simulink model "gm_uz_pmsm_model_9ph_21b_all_double_vnl"  (R2021b)
settings: Solver=FixedStepDiscrete  StartTime=0.0  StopTime=0.8  RelTol=1e-3
PreLoadFcn:
  | uz_pmsm_model_9ph_init_parameter
undefined symbols (not defined in the file or in its folder): a, b, c, friction_coefficient, inertia, k_i_d, k_i_q, k_p_d, k_p_q, Kpd, L_d, L_o1, L_o2, L_q, L_x1, L_x2, L_y1, L_y2, L_zero, polepair, psi_pm, R_1, static_friction_torque, Tnd, ts
libraries: hdlmdlgenlib x139, hdlsllib x90, dspsigops x21, simulink x17, slpidlib x2, spsAlphaBetaZerotodq0Lib x1, pid_lib x1, spsdq0toAlphaBetaZeroLib x1
(part 3 of 5)

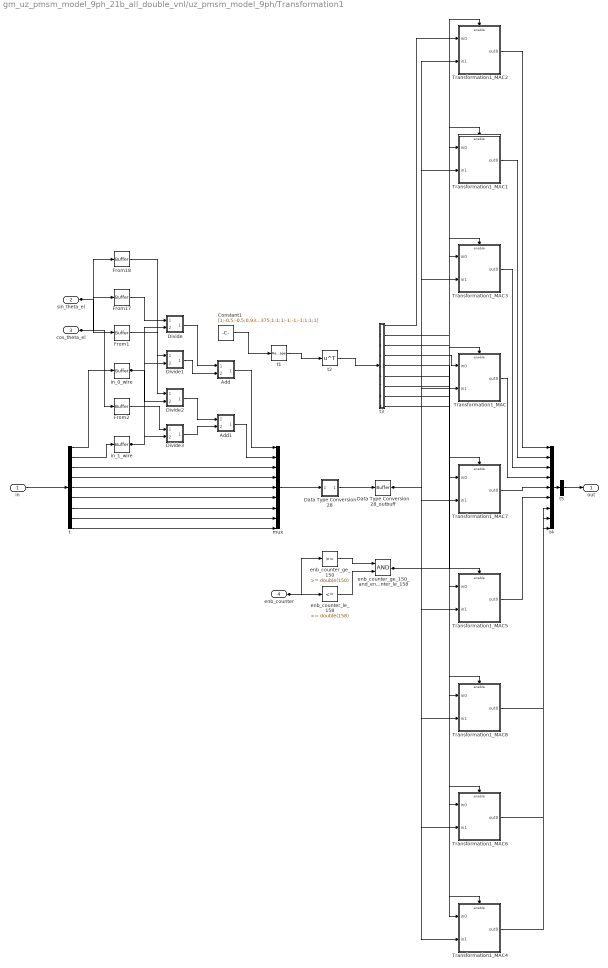
== system gm_uz_pmsm_model_9ph_21b_all_double_vnl/uz_pmsm_model_9ph/Transformation1 ==
  in : Inport  OutDataTypeStr=single  PortDimensions=[9]  SampleTime=1e-08
  sin_theta_el : Inport  Port=2  OutDataTypeStr=single  SampleTime=1e-08
  cos_theta_el : Inport  Port=3  OutDataTypeStr=single  SampleTime=1e-08
  enb_counter : Inport  Port=4  OutDataTypeStr=uint8  SampleTime=1e-08
  Add : Subsystem
      mask Display: disp('NFP\nadd');
  Add1 : Subsystem
      mask Display: disp('NFP\nadd');
  Constant1 : Constant  Value=[1;-0.5;-0.5;0.939697265625;-0.7660369873046875;-0.17364501953125;0.7660369873046875;-0.939697265625;0.17364501953125;0;0.86602783203125;-0.86602783203125;0.3420257568359375;0.642791748046875;-0.98480224609375;0.642791748046875;0.3420257568359375;-0.98480224609375;1;1;1;0.5;0.5;0.5;-0.5;-0.5;-0.5;0;0;0;0.86602783203125;0.86602783203125;0.86602783203125;0.86602783203125;0.86602783203125;0.86602783203125;1;-0.5;-0.5;-0.17364501953125;0.939697265625;-0.7660369873046875;-0.939697265625;0.17364501953125;0.7660369873046875;0;-0.86602783203125;0.86602783203125;0.98480224609375;-0.3420257568359375;-0.642791748046875;-0.3420257568359375;0.98480224609375;-0.642791748046875;1;-0.5;-0.5;-0.7660369873046875;-0.17364501953125;0.939697265625;0.17364501953125;0.7660369873046875;-0.939697265625;0;0.86602783203125;-0.86602783203125;0.642791748046875;-0.98480224609375;0.3420257568359375;-0.98480224609375;0.642791748046875;0.3420257568359375;1;1;1;-1;-1;-1;1;1;1]  OutDataTypeStr=fixdt(1, 18, 16)  SampleTime=1e-08
  Data Type Conversion28 : Subsystem
      mask Display: disp('NFP\nconv');
  Data Type Conversion28_outbuff : hdlmdlgenlib/Buffer
      settings: SourceProductBaseCode=SL
  Divide : Subsystem
      mask Display: disp('NFP\nmul');
  Divide1 : Subsystem
      mask Display: disp('NFP\nmul');
  Divide2 : Subsystem
      mask Display: disp('NFP\nmul');
  Divide3 : Subsystem
      mask Display: disp('NFP\nmul');
  From{1..2,17..18} (4 alike) : hdlmdlgenlib/Buffer
      settings: SourceProductBaseCode=SL
  Transformation1_MAC : Subsystem
      settings: MinAlgLoopOccurrences=on
  Transformation1_MAC1 : Subsystem
      settings: MinAlgLoopOccurrences=on
  Transformation1_MAC2 : Subsystem
      settings: MinAlgLoopOccurrences=on
  Transformation1_MAC3 : Subsystem
      settings: MinAlgLoopOccurrences=on
  Transformation1_MAC4 : Subsystem
      settings: MinAlgLoopOccurrences=on
  Transformation1_MAC5 : Subsystem
      settings: MinAlgLoopOccurrences=on
  Transformation1_MAC6 : Subsystem
      settings: MinAlgLoopOccurrences=on
  Transformation1_MAC7 : Subsystem
      settings: MinAlgLoopOccurrences=on
  Transformation1_MAC8 : Subsystem
      settings: MinAlgLoopOccurrences=on
  enb_counter_ge_150 : simulink/Logic and Bit Operations/Compare To Constant  relop=>=  const=double(150)  OutDataTypeStr=boolean
  enb_counter_ge_150_and_enb_counter_le_158 : Logic  AllPortsSameDT=off  OutDataTypeStr=boolean  SampleTime=1e-08
  enb_counter_le_158 : simulink/Logic and Bit Operations/Compare To Constant  relop=<=  const=double(158)  OutDataTypeStr=boolean
  in_0_wire : hdlmdlgenlib/Buffer
      settings: SourceProductBaseCode=SL
  in_1_wire : hdlmdlgenlib/Buffer
      settings: SourceProductBaseCode=SL
  mux : Mux  Inputs=9
  t : Demux  Outputs=9
  t1 : Reshape  OutputDimensionality=Customize  OutputDimensions=[9,9]
  t2 : Math  Operator=transpose  SaturateOnIntegerOverflow=on
  t3 : Subsystem
  t4 : Mux  Inputs=9
  t5 : Concatenate  NumInputs=1  Mode=Multidimensional array  ConcatenateDimension=2
  out : Outport  SampleTime=1e-08
  wires:
  enb_counter/1 -> enb_counter_ge_150/1, enb_counter_le_158/1
  cos_theta_el/1 -> From17/1, From2/1
  sin_theta_el/1 -> From1/1, From18/1
  in/1 -> t/1
  enb_counter_le_158/1 -> enb_counter_ge_150_and_enb_counter_le_158/2
  enb_counter_ge_150/1 -> enb_counter_ge_150_and_enb_counter_le_158/1
  enb_counter_ge_150_and_enb_counter_le_158/1 -> Transformation1_MAC4/Enable, Transformation1_MAC6/Enable, Transformation1_MAC8/Enable, Transformation1_MAC5/Enable, Transformation1_MAC7/Enable, Transformation1_MAC/Enable, Transformation1_MAC3/Enable, Transformation1_MAC1/Enable, Transformation1_MAC2/Enable
  t3/9(out8) -> Transformation1_MAC4/1(in0)
  t3/8(out7) -> Transformation1_MAC6/1(in0)
  t3/7(out6) -> Transformation1_MAC8/1(in0)
  t3/6(out5) -> Transformation1_MAC5/1(in0)
  t3/5(out4) -> Transformation1_MAC7/1(in0)
  t3/4(out3) -> Transformation1_MAC/1(in0)
  t3/3(out2) -> Transformation1_MAC3/1(in0)
  t3/2(out1) -> Transformation1_MAC1/1(in0)
  t3/1(out0) -> Transformation1_MAC2/1(in0)
  Divide3/1(Out1) -> Add1/2(In2)
  Divide2/1(Out1) -> Add1/1(In1)
  Divide1/1(Out1) -> Add/2(In2)
  Divide/1(Out1) -> Add/1(In1)
  Data Type Conversion28/1(Out1) -> Data Type Conversion28_outbuff/1
  Add1/1(Out1) -> mux/2
  Add/1(Out1) -> mux/1
  t4/1 -> t5/1
  Transformation1_MAC4/1(out0) -> t4/9
  Transformation1_MAC6/1(out0) -> t4/8
  Transformation1_MAC8/1(out0) -> t4/7
  Transformation1_MAC5/1(out0) -> t4/6
  Transformation1_MAC7/1(out0) -> t4/5
  Transformation1_MAC/1(out0) -> t4/4
  Transformation1_MAC3/1(out0) -> t4/3
  Transformation1_MAC1/1(out0) -> t4/2
  Transformation1_MAC2/1(out0) -> t4/1
  t2/1 -> t3/1(in0)
  Constant1/1 -> t1/1
  t/9 -> mux/9
  t/8 -> mux/8
  t/7 -> mux/7
  t/6 -> mux/6
  t/5 -> mux/5
  t/4 -> mux/4
  t/3 -> mux/3
  t/2 -> in_1_wire/1
  t/1 -> in_0_wire/1
  mux/1 -> Data Type Conversion28/1(In1)
  t5/1 -> out/1
  From2/1 -> Divide3/1(In1)
  From18/1 -> Divide1/1(In1)
  From17/1 -> Divide/1(In1)
  From1/1 -> Divide2/1(In1)
  in_1_wire/1 -> Divide1/2(In2), Divide3/2(In2)
  in_0_wire/1 -> Divide/2(In2), Divide2/2(In2)
  Data Type Conversion28_outbuff/1 -> Transformation1_MAC4/2(in1), Transformation1_MAC6/2(in1), Transformation1_MAC8/2(in1), Transformation1_MAC5/2(in1), Transformation1_MAC7/2(in1), Transformation1_MAC/2(in1), Transformation1_MAC3/2(in1), Transformation1_MAC1/2(in1), Transformation1_MAC2/2(in1)
  t1/1 -> t2/1

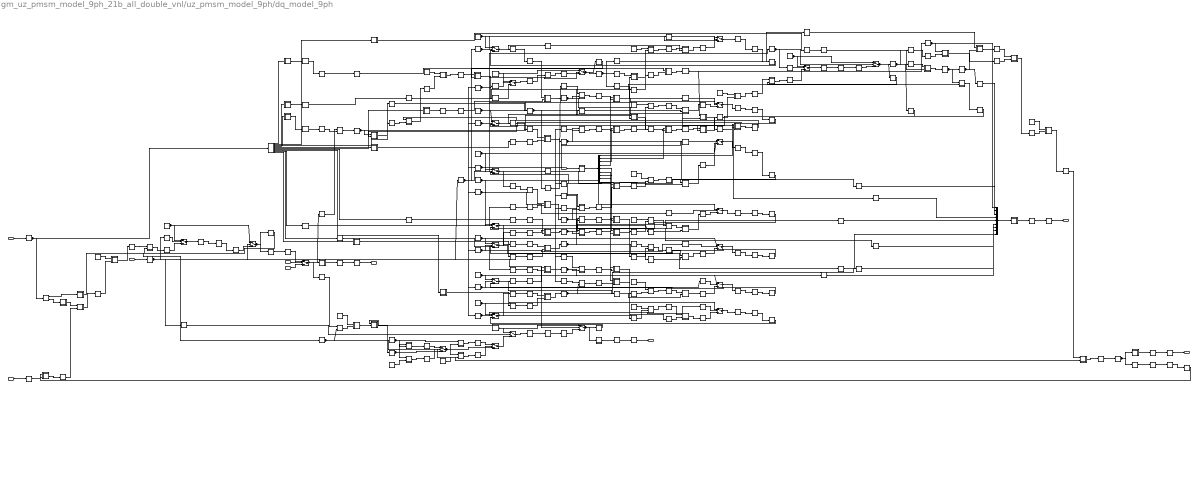
== system gm_uz_pmsm_model_9ph_21b_all_double_vnl/uz_pmsm_model_9ph/dq_model_9ph ==
  note: This signal introduces an algebraic loop if simulate_mechanical is true!
  note: PMSM electric and magentic
  note: Mechanical
  note: o1 equation
  note: DQ equations
  note: o2 equation
  note: x1 equation
  note: y1 equation
  note: x2 equation
  note: y2 equation
  note: zero equation
  note: load torque negative!!!
  note: https://de.mathworks.com/help/releases/R2021a/hdlcoder/ug/troubleshoot-generate-implementation-model-from-simscape-pmsm.html?searchHighlight=troubleshoot-generate-implementation-model-from-simscape-pmsm&s_tid=doc_srchtitle
  load_torque : Inport  OutDataTypeStr=single  PortDimensions=1  SampleTime=1e-08
  <reset_integrators> : Inport  Port=2  OutDataTypeStr=boolean  PortDimensions=1  SampleTime=1e-08
  <simulate_mechanical> : Inport  Port=3  OutDataTypeStr=boolean  PortDimensions=1  SampleTime=1e-08
  omega_mech : Inport  Port=4  OutDataTypeStr=single  PortDimensions=1  SampleTime=1e-08
  voltage_input_dq : Inport  Port=5  OutDataTypeStr=single  PortDimensions=[9]  SampleTime=1e-08
  physical_parameters : Inport  Port=6  SampleTime=2e-06
  Add : Subsystem
      mask Display: disp('NFP\nadd');
  Add1 : Subsystem
      mask Display: disp('NFP\nadd');
  Add1_outbuff : hdlmdlgenlib/Buffer
      settings: SourceProductBaseCode=SL
  Add2 : Subsystem
      mask Display: disp('NFP\nadd');
  Add2_outbuff : hdlmdlgenlib/Buffer
      settings: SourceProductBaseCode=SL
  Add3 : Subsystem
      mask Display: disp('NFP\nadd');
  Add3_outbuff : hdlmdlgenlib/Buffer
      settings: SourceProductBaseCode=SL
  Add4 : Subsystem
      mask Display: disp('NFP\nadd');
  Add4_outbuff : hdlmdlgenlib/Buffer
      settings: SourceProductBaseCode=SL
  Add5 : Subsystem
      mask Display: disp('NFP\nadd');
  Add5_outbuff : hdlmdlgenlib/Buffer
      settings: SourceProductBaseCode=SL
  Add6 : Subsystem
      mask Display: disp('NFP\nadd');
  Add6_outbuff : hdlmdlgenlib/Buffer
      settings: SourceProductBaseCode=SL
  Add_outbuff : hdlmdlgenlib/Buffer
      settings: SourceProductBaseCode=SL
  Compare To Constant1_const : Constant  Value=double(-3.1415927410125732)  OutDataTypeStr=double  SampleTime=1e-08
  Compare To Constant1_relop : Subsystem
      mask Display: disp('NFP\nrelop');
  Compare To Constant1_relop_outbuff : hdlmdlgenlib/Buffer
      settings: SourceProductBaseCode=SL
  Compare To Constant_const : Constant  Value=double(3.1415927410125732)  OutDataTypeStr=double  SampleTime=1e-08
  Compare To Constant_relop : Subsystem
      mask Display: disp('NFP\nrelop');
  Compare To Constant_relop_outbuff : hdlmdlgenlib/Buffer
      settings: SourceProductBaseCode=SL
  Constant : Constant  Value=double(6.283185307179586)  OutDataTypeStr=double  SampleTime=1e-08
  Data Type Conversion : Subsystem
      mask Display: disp('NFP\nconv');
  Data Type Conversion1 : Subsystem
      mask Display: disp('NFP\nconv');
  Data Type Conversion10 : Subsystem
      mask Display: disp('NFP\nconv');
  Data Type Conversion11 : Subsystem
      mask Display: disp('NFP\nconv');
  Data Type Conversion12 : Subsystem
      mask Display: disp('NFP\nconv');
  Data Type Conversion13 : Subsystem
      mask Display: disp('NFP\nconv');
  Data Type Conversion1_outbuff : hdlmdlgenlib/Buffer
      settings: SourceProductBaseCode=SL
  Data Type Conversion2 : Subsystem
      mask Display: disp('NFP\nconv');
  Data Type Conversion21 : Subsystem
      mask Display: disp('NFP\nconv');
  Data Type Conversion3 : Subsystem
      mask Display: disp('NFP\nconv');
  Data Type Conversion31 : Subsystem
      mask Display: disp('NFP\nconv');
  Data Type Conversion4 : Subsystem
      mask Display: disp('NFP\nconv');
  Data Type Conversion41 : Subsystem
      mask Display: disp('NFP\nconv');
  Data Type Conversion4_outbuff : hdlmdlgenlib/Buffer
      settings: SourceProductBaseCode=SL
  Data Type Conversion5 : Subsystem
      mask Display: disp('NFP\nconv');
  Data Type Conversion51 : Subsystem
      mask Display: disp('NFP\nconv');
  Data Type Conversion6 : Subsystem
      mask Display: disp('NFP\nconv');
  Data Type Conversion61 : Subsystem
      mask Display: disp('NFP\nconv');
  Data Type Conversion7 : Subsystem
      mask Display: disp('NFP\nconv');
  Data Type Conversion71 : Subsystem
      mask Display: disp('NFP\nconv');
  Data Type Conversion8 : Subsystem
      mask Display: disp('NFP\nconv');
  Data Type Conversion9 : Subsystem
      mask Display: disp('NFP\nconv');
  Delay : RateTransition  OutPortSampleTimeOpt=Multiple of input port sample time  OutPortSampleTimeMultiple=200
  Delay1 : RateTransition  OutPortSampleTimeOpt=Multiple of input port sample time  OutPortSampleTimeMultiple=200
  Delay1_lowered{,1..10} (11 alike) : RateTransition  OutPortSampleTimeOpt=Multiple of input port sample time  OutPortSampleTimeMultiple=200
  Delay2 : RateTransition  OutPortSampleTimeOpt=Multiple of input port sample time  OutPortSampleTimeMultiple=200
  Divide : Subsystem
      mask Display: disp('NFP\nmul');
  Divide1 : Subsystem
      mask Display: disp('NFP\nmul');
  Divide10 : Subsystem
      mask Display: disp('NFP\nmul');
  Divide10_outbuff : hdlmdlgenlib/Buffer
      settings: SourceProductBaseCode=SL
  Divide11 : Subsystem
      mask Display: disp('NFP\nmul');
  Divide11_outbuff : hdlmdlgenlib/Buffer
      settings: SourceProductBaseCode=SL
  Divide12 : Subsystem
      mask Display: disp('NFP\nmul');
  Divide12_outbuff : hdlmdlgenlib/Buffer
      settings: SourceProductBaseCode=SL
  Divide13 : Subsystem
      mask Display: disp('NFP\nmul');
  Divide13_outbuff : hdlmdlgenlib/Buffer
      settings: SourceProductBaseCode=SL
  Divide1_outbuff : hdlmdlgenlib/Buffer
      settings: SourceProductBaseCode=SL
  Divide2 : Subsystem
      mask Display: disp('NFP\nmul');
  Divide2_outbuff : hdlmdlgenlib/Buffer
      settings: SourceProductBaseCode=SL
  Divide3 : Subsystem
      mask Display: disp('NFP\nmul');
  Divide3_outbuff : hdlmdlgenlib/Buffer
      settings: SourceProductBaseCode=SL
  Divide4 : Subsystem
      mask Display: disp('NFP\nmul');
  Divide4_outbuff : hdlmdlgenlib/Buffer
      settings: SourceProductBaseCode=SL
  Divide5 : Subsystem
      mask Display: disp('NFP\nmul');
  Divide5_outbuff : hdlmdlgenlib/Buffer
      settings: SourceProductBaseCode=SL
  Divide6 : Subsystem
      mask Display: disp('NFP\nmul');
  Divide6_outbuff : hdlmdlgenlib/Buffer
      settings: SourceProductBaseCode=SL
  Divide7 : Subsystem
      mask Display: disp('NFP\nmul');
  Divide7_outbuff : hdlmdlgenlib/Buffer
      settings: SourceProductBaseCode=SL
  Divide8 : Subsystem
      mask Display: disp('NFP\nmul');
  Divide8_outbuff : hdlmdlgenlib/Buffer
      settings: SourceProductBaseCode=SL
  Divide9 : Subsystem
      mask Display: disp('NFP\nmul');
  Divide9_outbuff : hdlmdlgenlib/Buffer
      settings: SourceProductBaseCode=SL
  Divide_outbuff : hdlmdlgenlib/Buffer
      settings: SourceProductBaseCode=SL
  Factor : Subsystem
      mask Display: disp('NFP\nmul');
  Factor_const : Constant  Value=double(4.5)  OutDataTypeStr=double  SampleTime=1e-08
  Factor_outbuff : hdlmdlgenlib/Buffer
      settings: SourceProductBaseCode=SL
  From{2..24,26..27,30..31} (27 alike) : hdlmdlgenlib/Buffer
      settings: SourceProductBaseCode=SL
  Gain : Subsystem
      mask Display: disp('NFP\nmul');
  Gain1 : Subsystem
      mask Display: disp('NFP\nmul');
  Gain10 : Subsystem
      mask Display: disp('NFP\nmul');
  Gain2 : Subsystem
      mask Display: disp('NFP\nmul');
  Gain3 : Subsystem
      mask Display: disp('NFP\nmul');
  Gain4 : Subsystem
      mask Display: disp('NFP\nmul');
  Gain5 : Subsystem
      mask Display: disp('NFP\nmul');
  Gain6 : Subsystem
      mask Display: disp('NFP\nmul');
  Gain7 : Subsystem
      mask Display: disp('NFP\nmul');
  Gain8 : Subsystem
      mask Display: disp('NFP\nmul');
  Gain9 : Subsystem
      mask Display: disp('NFP\nmul');
  Gain_const{,1..10} (11 alike) : Constant  Value=double(2e-06)  OutDataTypeStr=double  SampleTime=1e-08
  Gain_outbuff{,1..9} (10 alike) : hdlmdlgenlib/Buffer
      settings: SourceProductBaseCode=SL
  Goto{1,9..15,32..36} (13 alike) : hdlmdlgenlib/Buffer
      settings: SourceProductBaseCode=SL
  Initial_Val{,1..10} (11 alike) : Constant  Value=double(0)  OutDataTypeStr=double  SampleTime=1e-08
  M_Mi1 : hdlmdlgenlib/Buffer
      settings: SourceProductBaseCode=SL
  Product : Subsystem
      mask Display: disp('NFP\nmul');
  Product1 : Subsystem
      mask Display: disp('NFP\nmul');
  Product10 : Subsystem
      mask Display: disp('NFP\nmul');
  Product10_outbuff : hdlmdlgenlib/Buffer
      settings: SourceProductBaseCode=SL
  Product11 : Subsystem
      mask Display: disp('NFP\nmul');
  Product11_outbuff : hdlmdlgenlib/Buffer
      settings: SourceProductBaseCode=SL
  Product1_outbuff : hdlmdlgenlib/Buffer
      settings: SourceProductBaseCode=SL
  Product2 : Subsystem
      mask Display: disp('NFP\nmul');
  Product2_outbuff : hdlmdlgenlib/Buffer
      settings: SourceProductBaseCode=SL
  Product3 : Subsystem
      mask Display: disp('NFP\nmul');
  Product3_outbuff : hdlmdlgenlib/Buffer
      settings: SourceProductBaseCode=SL
  Product4 : Subsystem
      mask Display: disp('NFP\nmul');
  Product5 : Subsystem
      mask Display: disp('NFP\nmul');
  Product5_outbuff : hdlmdlgenlib/Buffer
      settings: SourceProductBaseCode=SL
  Product6 : Subsystem
      mask Display: disp('NFP\nmul');
  Product6_outbuff : hdlmdlgenlib/Buffer
      settings: SourceProductBaseCode=SL
  Product7 : Subsystem
      mask Display: disp('NFP\nmul');
  Product7_outbuff : hdlmdlgenlib/Buffer
      settings: SourceProductBaseCode=SL
  Product8 : Subsystem
      mask Display: disp('NFP\nmul');
  Product8_outbuff : hdlmdlgenlib/Buffer
      settings: SourceProductBaseCode=SL
  Product9 : Subsystem
      mask Display: disp('NFP\nmul');
  Product9_outbuff : hdlmdlgenlib/Buffer
      settings: SourceProductBaseCode=SL
  Product_outbuff : hdlmdlgenlib/Buffer
      settings: SourceProductBaseCode=SL
  Sum : Subsystem
      mask Display: disp('NFP\nadd');
  Sum1 : Subsystem
      mask Display: disp('NFP\nadd');
  Sum11 : Subsystem
      mask Display: disp('NFP\nadd');
  Sum1_outbuff : hdlmdlgenlib/Buffer
      settings: SourceProductBaseCode=SL
  Sum1_outbuff1 : hdlmdlgenlib/Buffer
      settings: SourceProductBaseCode=SL
  Sum1_stage2 : Subsystem
      mask Display: disp('NFP\nadd');
  Sum1_stage2_outbuff : hdlmdlgenlib/Buffer
      settings: SourceProductBaseCode=SL
  Sum1_stage3 : Subsystem
      mask Display: disp('NFP\nadd');
  Sum1_stage3_outbuff : hdlmdlgenlib/Buffer
      settings: SourceProductBaseCode=SL
  Sum2 : Subsystem
      mask Display: disp('NFP\nadd');
  Sum21 : Subsystem
      mask Display: disp('NFP\nadd');
  Sum2_outbuff : hdlmdlgenlib/Buffer
      settings: SourceProductBaseCode=SL
  Sum2_outbuff1 : hdlmdlgenlib/Buffer
      settings: SourceProductBaseCode=SL
  Sum3 : Subsystem
      mask Display: disp('NFP\nadd');
  Sum31 : Subsystem
      mask Display: disp('NFP\nadd');
  Sum310 : Subsystem
      mask Display: disp('NFP\nadd');
  Sum32 : Subsystem
      mask Display: disp('NFP\nadd');
  Sum33 : Subsystem
      mask Display: disp('NFP\nadd');
  Sum34 : Subsystem
      mask Display: disp('NFP\nadd');
  Sum35 : Subsystem
      mask Display: disp('NFP\nadd');
  Sum36 : Subsystem
      mask Display: disp('NFP\nadd');
  Sum37 : Subsystem
      mask Display: disp('NFP\nadd');
  Sum38 : Subsystem
      mask Display: disp('NFP\nadd');
  Sum39 : Subsystem
      mask Display: disp('NFP\nadd');
  Sum3_outbuff{,1..10} (11 alike) : hdlmdlgenlib/Buffer
      settings: SourceProductBaseCode=SL
  Sum_outbuff : hdlmdlgenlib/Buffer
      settings: SourceProductBaseCode=SL
  Sum_stage2 : Subsystem
      mask Display: disp('NFP\nadd');
  Sum_stage2_outbuff : hdlmdlgenlib/Buffer
      settings: SourceProductBaseCode=SL
  Sum_stage3 : Subsystem
      mask Display: disp('NFP\nadd');
  Sum_stage3_outbuff : hdlmdlgenlib/Buffer
      settings: SourceProductBaseCode=SL
  Switch : Switch  Criteria=u2 ~= 0  Threshold=double(0)  OutDataTypeStr=double  SampleTime=1e-08
  Switch1 : Switch  Criteria=u2 ~= 0  Threshold=double(0)  OutDataTypeStr=double  SampleTime=1e-08
  Switch11 : Switch  Criteria=u2 ~= 0  Threshold=double(0)  OutDataTypeStr=double  SampleTime=1e-08
  bus_selector : BusSelector  OutputSignals=1_L_d,1_L_q,R_1,polepair,psi_pm,L_z1,L_z2,L_x1,L_y1,L_x2,L_y2,L_z3
  bus_selector1 : BusSelector  OutputSignals=polepair,1_J
  crp_out_delay{,1..13} (14 alike) : Delay  DelayLength=double(1)  InitialCondition=0  SampleTime=1e-08
  delayMatch{,1..3,5..7,10..11,27..46} (29 alike) : Delay  DelayLength=double(1)  InitialCondition=0  SampleTime=1e-08
  delayMatch{4,8,12..18} (9 alike) : Delay  DelayLength=double(3)  InitialCondition=0  SampleTime=1e-08
  delayMatch{9,19..26} (9 alike) : Delay  DelayLength=double(6)  InitialCondition=0  SampleTime=1e-08
  delayMatch47 : Delay  DelayLength=double(42)  InitialCondition=0  SampleTime=1e-08
  delayMatch48 : Delay  DelayLength=double(27)  InitialCondition=0  SampleTime=1e-08
  delayMatch49 : Delay  DelayLength=double(87)  InitialCondition=0  SampleTime=1e-08
  delayMatch50 : Delay  DelayLength=double(87)  InitialCondition=0  SampleTime=1e-08
  i_d : hdlmdlgenlib/Buffer
      settings: SourceProductBaseCode=SL
  i_q : hdlmdlgenlib/Buffer
      settings: SourceProductBaseCode=SL
  in0_buff : hdlmdlgenlib/Buffer
      settings: SourceProductBaseCode=SL
  in10_repeat : RateTransition  Integrity=off  Deterministic=off  OutPortSampleTimeOpt=Multiple of input port sample time  OutPortSampleTimeMultiple=1/200
  in11_repeat : dspsigops/Repeat  N=double(200)  RateOptions=Allow multirate processing  ic=0  mode=Unused parameter value
  in12_repeat : dspsigops/Repeat  N=double(200)  RateOptions=Allow multirate processing  ic=0  mode=Unused parameter value
  in13_repeat : dspsigops/Repeat  N=double(200)  RateOptions=Allow multirate processing  ic=0  mode=Unused parameter value
  in15_repeat : dspsigops/Repeat  N=double(200)  RateOptions=Allow multirate processing  ic=0  mode=Unused parameter value
  in1_repeat : dspsigops/Repeat  N=double(200)  RateOptions=Allow multirate processing  ic=0  mode=Unused parameter value
  in2_repeat : dspsigops/Repeat  N=double(200)  RateOptions=Allow multirate processing  ic=0  mode=Unused parameter value
  in3_repeat : dspsigops/Repeat  N=double(200)  RateOptions=Allow multirate processing  ic=0  mode=Unused parameter value
  in4_repeat : dspsigops/Repeat  N=double(200)  RateOptions=Allow multirate processing  ic=0  mode=Unused parameter value
  in5_repeat : dspsigops/Repeat  N=double(200)  RateOptions=Allow multirate processing  ic=0  mode=Unused parameter value
  in6_repeat : dspsigops/Repeat  N=double(200)  RateOptions=Allow multirate processing  ic=0  mode=Unused parameter value
  in8_repeat : dspsigops/Repeat  N=double(200)  RateOptions=Allow multirate processing  ic=0  mode=Unused parameter value
  in9_repeat : dspsigops/Repeat  N=double(200)  RateOptions=Allow multirate processing  ic=0  mode=Unused parameter value
  integrator_out1 : hdlmdlgenlib/Buffer
      settings: SourceProductBaseCode=SL
  mechanical_system_out1 : hdlmdlgenlib/Buffer
      settings: SourceProductBaseCode=SL
  mux : Mux  Inputs=9
  pmsm_out1 : hdlmdlgenlib/Buffer
      settings: SourceProductBaseCode=SL
  pmsm_out2 : hdlmdlgenlib/Buffer
      settings: SourceProductBaseCode=SL
  psi_{,1..6} (7 alike) : hdlmdlgenlib/Buffer
      settings: SourceProductBaseCode=SL
  psi_d : hdlmdlgenlib/Buffer
      settings: SourceProductBaseCode=SL
  psi_q : hdlmdlgenlib/Buffer
      settings: SourceProductBaseCode=SL
  reset_in{,1..10} (11 alike) : Switch  Criteria=u2 ~= 0  Threshold=double(0)  OutDataTypeStr=double  SampleTime=1e-08
  reset_out{,1..10} (11 alike) : Switch  Criteria=u2 ~= 0  Threshold=double(0)  OutDataTypeStr=double  SampleTime=1e-08
  t : Demux  Outputs=9
  theta_el : Outport  SampleTime=1e-08
  currents_dq_output : Outport  Port=2  SampleTime=1e-08
  M_Mi : Outport  Port=3  SampleTime=2e-06
  omega_out : Outport  Port=4  SampleTime=2e-06
  wires:
  delayMatch48/1 -> delayMatch50/1
  delayMatch47/1 -> delayMatch49/1
  delayMatch43/1 -> reset_in6/2
  delayMatch42/1 -> Sum35/2(In2)
  Divide10_outbuff/1 -> Add5/2(In2)
  delayMatch41/1 -> reset_in5/2
  delayMatch40/1 -> Sum34/2(In2)
  Divide8_outbuff/1 -> Add4/2(In2)
  delayMatch39/1 -> reset_in4/2
  delayMatch38/1 -> Sum33/2(In2)
  Divide6_outbuff/1 -> Add3/2(In2)
  delayMatch37/1 -> reset_in3/2
  delayMatch36/1 -> Sum32/2(In2)
  Divide4_outbuff/1 -> Add2/2(In2)
  delayMatch35/1 -> reset_in2/2
  delayMatch34/1 -> Sum31/2(In2)
  Product8_outbuff/1 -> Sum_stage2/2(In2)
  delayMatch32/1 -> reset_in1/2
  delayMatch31/1 -> Sum3/2(In2)
  Divide12_outbuff/1 -> Add6/2(In2)
  delayMatch30/1 -> reset_in7/2
  delayMatch29/1 -> Sum36/2(In2)
  Divide_outbuff/1 -> Add/2(In2)
  delayMatch28/1 -> reset_in8/2
  delayMatch27/1 -> Sum37/2(In2)
  Divide2_outbuff/1 -> Add1/2(In2)
  delayMatch7/1 -> reset_in9/2
  delayMatch6/1 -> Sum39/2(In2)
  Product1_outbuff/1 -> Sum1_stage2/2(In2)
  reset_in10/1 -> crp_out_delay13/1
  reset_in6/1 -> crp_out_delay12/1
  reset_in5/1 -> crp_out_delay11/1
  reset_in4/1 -> crp_out_delay10/1
  reset_in3/1 -> crp_out_delay9/1
  reset_in1/1 -> crp_out_delay7/1
  reset_in7/1 -> crp_out_delay6/1
  reset_in8/1 -> crp_out_delay5/1
  M_Mi1/1 -> crp_out_delay4/1, Data Type Conversion4/1(In1)
  reset_in9/1 -> crp_out_delay2/1
  reset_in/1 -> crp_out_delay/1
  reset_out10/1 -> integrator_out1/1, delayMatch45/1
  From27/1 -> reset_out5/2, delayMatch43/1
  reset_out5/1 -> psi_4/1, delayMatch42/1
  From26/1 -> Divide10/1(In1)
  From23/1 -> reset_out4/2, delayMatch41/1
  reset_out4/1 -> psi_3/1, delayMatch40/1
  From22/1 -> Divide8/1(In1)
  From19/1 -> reset_out3/2, delayMatch39/1
  reset_out3/1 -> psi_2/1, delayMatch38/1
  From18/1 -> Divide6/1(In1)
  From15/1 -> reset_out2/2, delayMatch37/1
  reset_out2/1 -> psi_1/1, delayMatch36/1
  From14/1 -> Divide4/1(In1)
  From2/1 -> reset_out1/2, delayMatch35/1
  reset_out1/1 -> psi_d/1, delayMatch34/1
  Product_outbuff/1 -> Sum_stage3/2(In2)
  psi_q/1 -> pmsm_out2/1, delayMatch4/1, delayMatch33/1
  Data Type Conversion4_outbuff/1 -> Product7/2(In2), Product8/2(In2), Goto32/1
  From31/1 -> reset_out6/2, delayMatch32/1
  reset_out6/1 -> psi_5/1, delayMatch31/1
  From30/1 -> Divide12/1(In1)
  From5/1 -> reset_out7/2, delayMatch30/1
  reset_out7/1 -> psi_/1, delayMatch29/1
  From4/1 -> Divide/1(In1)
  From9/1 -> reset_out8/2, delayMatch28/1
  reset_out8/1 -> psi_6/1, delayMatch27/1
  From8/1 -> Divide2/1(In1)
  i_q/1 -> Product3/2(In2), delayMatch19/1
  psi_5/1 -> delayMatch18/1
  psi_4/1 -> delayMatch17/1
  psi_3/1 -> delayMatch16/1
  psi_2/1 -> delayMatch15/1
  psi_1/1 -> delayMatch14/1
  psi_6/1 -> delayMatch13/1
  psi_/1 -> delayMatch12/1
  Data Type Conversion1_outbuff/1 -> Product9/2(In2), Product4/2(In2)
  Product3_outbuff/1 -> Sum38/1(In1)
  pmsm_out2/1 -> delayMatch11/1
  pmsm_out1/1 -> delayMatch10/1
  From10/1 -> delayMatch9/1
  psi_d/1 -> pmsm_out1/1, delayMatch5/1, delayMatch8/1
  From3/1 -> reset_out9/2, delayMatch7/1
  reset_out9/1 -> psi_q/1, delayMatch6/1
  Product7_outbuff/1 -> Sum1_stage3/2(In2)
  delayMatch8/1 -> Sum21/1(In1)
  delayMatch33/1 -> Product/2(In2)
  Switch11/1 -> Data Type Conversion5/1(In1), delayMatch/1, delayMatch3/1
  delayMatch46/1 -> reset_in10/2
  Switch/1 -> Switch1/3, Compare To Constant1_relop/1(In1), Sum2/2(In2)
  Compare To Constant1_relop_outbuff/1 -> Switch1/2
  Sum_outbuff/1 -> Switch/3, Sum1/1(In1), Compare To Constant_relop/1(In1)
  Compare To Constant_relop_outbuff/1 -> Switch/2
  reset_out/1 -> Data Type Conversion6/1(In1), delayMatch1/1
  delayMatch3/1 -> Product10/1(In1)
  in0_buff/1 -> reset_out10/2, reset_out/2, Goto1/1, delayMatch2/1, delayMatch46/1
  Gain10/1(Out1) -> Gain_outbuff9/1
  Gain9/1(Out1) -> Gain_outbuff8/1
  Gain8/1(Out1) -> Gain_outbuff7/1
  Gain7/1(Out1) -> Gain_outbuff6/1
  Gain6/1(Out1) -> Gain_outbuff5/1
  Gain5/1(Out1) -> Gain_outbuff4/1
  Gain4/1(Out1) -> Gain_outbuff3/1
  Gain3/1(Out1) -> Gain_outbuff2/1
  Gain2/1(Out1) -> Gain_outbuff1/1
  Gain1/1(Out1) -> Gain_outbuff/1
  Factor/1(Out1) -> Factor_outbuff/1
  Gain/1(Out1) -> Sum/2(In2)
  Data Type Conversion13/1(Out1) -> Data Type Conversion1_outbuff/1
  Product4/1(Out1) -> Gain/2(In2)
  Sum310/1(Out1) -> Sum3_outbuff10/1
  Product11/1(Out1) -> Product11_outbuff/1
  Sum11/1(Out1) -> Sum1_outbuff1/1
  Data Type Conversion71/1(Out1) -> Sum11/2(In2)
  Data Type Conversion21/1(Out1) -> Product11/1(In1)
  Product10/1(Out1) -> Product10_outbuff/1
  Product1/1(Out1) -> Product1_outbuff/1
  Sum1_stage3/1(Out1) -> Sum1_stage3_outbuff/1
  Sum1_stage2/1(Out1) -> Sum1_stage2_outbuff/1
  Sum39/1(Out1) -> Sum3_outbuff9/1
  Product2/1(Out1) -> Product2_outbuff/1
  Sum38/1(Out1) -> Sum3_outbuff8/1
  Product3/1(Out1) -> Product3_outbuff/1
  Sum21/1(Out1) -> Sum2_outbuff1/1
  Product5/1(Out1) -> Product5_outbuff/1
  Product6/1(Out1) -> Product6_outbuff/1
  Product7/1(Out1) -> Product7_outbuff/1
  Data Type Conversion41/1(Out1) -> Data Type Conversion4_outbuff/1
  Divide2/1(Out1) -> Divide2_outbuff/1
  Add1/1(Out1) -> Add1_outbuff/1
  Sum37/1(Out1) -> Sum3_outbuff7/1
  Divide3/1(Out1) -> Divide3_outbuff/1
  Data Type Conversion8/1(Out1) -> Goto10/1
  Data Type Conversion7/1(Out1) -> Goto9/1
  Divide1/1(Out1) -> Divide1_outbuff/1
  Divide/1(Out1) -> Divide_outbuff/1
  Add/1(Out1) -> Add_outbuff/1
  Sum36/1(Out1) -> Sum3_outbuff6/1
  Divide13/1(Out1) -> Divide13_outbuff/1
  Data Type Conversion31/1(Out1) -> Goto15/1
  Divide12/1(Out1) -> Divide12_outbuff/1
  Add6/1(Out1) -> Add6_outbuff/1
  Data Type Conversion/1(Out1) -> t/1
  Add5/1(Out1) -> Add5_outbuff/1
  Sum35/1(Out1) -> Sum3_outbuff5/1
  Divide11/1(Out1) -> Divide11_outbuff/1
  Data Type Conversion12/1(Out1) -> Goto14/1
  Divide10/1(Out1) -> Divide10_outbuff/1
  Add4/1(Out1) -> Add4_outbuff/1
  Sum34/1(Out1) -> Sum3_outbuff4/1
  Divide9/1(Out1) -> Divide9_outbuff/1
  Data Type Conversion11/1(Out1) -> Goto13/1
  Divide8/1(Out1) -> Divide8_outbuff/1
  Add3/1(Out1) -> Add3_outbuff/1
  Sum33/1(Out1) -> Sum3_outbuff3/1
  Divide7/1(Out1) -> Divide7_outbuff/1
  Data Type Conversion10/1(Out1) -> Goto12/1
  Divide6/1(Out1) -> Divide6_outbuff/1
  Add2/1(Out1) -> Add2_outbuff/1
  Sum32/1(Out1) -> Sum3_outbuff2/1
  Divide5/1(Out1) -> Divide5_outbuff/1
  Data Type Conversion9/1(Out1) -> Goto11/1
  Divide4/1(Out1) -> Divide4_outbuff/1
  Sum_stage3/1(Out1) -> Sum_stage3_outbuff/1
  Sum_stage2/1(Out1) -> Sum_stage2_outbuff/1
  Product/1(Out1) -> Product_outbuff/1
  Product8/1(Out1) -> Product8_outbuff/1
  Sum31/1(Out1) -> Sum3_outbuff1/1
  Sum3/1(Out1) -> Sum3_outbuff/1
  Data Type Conversion61/1(Out1) -> Goto33/1
  Data Type Conversion51/1(Out1) -> Goto34/1
  Data Type Conversion2/1(Out1) -> Goto35/1
  Data Type Conversion1/1(Out1) -> Goto36/1
  Data Type Conversion3/1(Out1) -> delayMatch48/1
  Product9/1(Out1) -> Product9_outbuff/1
  Data Type Conversion4/1(Out1) -> crp_out_delay3/1
  Data Type Conversion5/1(Out1) -> crp_out_delay1/1
  Sum/1(Out1) -> Sum_outbuff/1
  Compare To Constant_relop/1(Out1) -> Compare To Constant_relop_outbuff/1
  Sum2/1(Out1) -> Sum2_outbuff/1
  Sum1/1(Out1) -> Sum1_outbuff/1
  Compare To Constant1_relop/1(Out1) -> Compare To Constant1_relop_outbuff/1
  Data Type Conversion6/1(Out1) -> delayMatch47/1
  delayMatch44/1 -> Sum11/1(In1)
  delayMatch2/1 -> reset_in/2
  Gain_const10/1 -> Gain10/1(In1)
  Gain_const9/1 -> Gain9/1(In1)
  Gain_const8/1 -> Gain8/1(In1)
  Gain_const7/1 -> Gain7/1(In1)
  Gain_const6/1 -> Gain6/1(In1)
  Gain_const5/1 -> Gain5/1(In1)
  Gain_const4/1 -> Gain4/1(In1)
  Gain_const3/1 -> Gain3/1(In1)
  Gain_const2/1 -> Gain2/1(In1)
  Gain_const1/1 -> Gain1/1(In1)
  Factor_const/1 -> Factor/1(In1)
  Gain_const/1 -> Gain/1(In1)
  Sum1_stage2_outbuff/1 -> Sum1_stage3/1(In1)
  t/9 -> Add6/1(In1)
  t/8 -> Add5/1(In1)
  t/7 -> Add4/1(In1)
  t/6 -> Add3/1(In1)
  t/5 -> Add2/1(In1)
  t/4 -> Add1/1(In1)
  t/3 -> Add/1(In1)
  t/2 -> Sum1_stage2/1(In1)
  t/1 -> Sum_stage2/1(In1)
  Sum_stage2_outbuff/1 -> Sum_stage3/1(In1)
  Compare To Constant_const/1 -> Compare To Constant_relop/2(In2)
  Compare To Constant1_const/1 -> Compare To Constant1_relop/2(In2)
  reset_in2/1 -> crp_out_delay8/1
  bus_selector1/2 -> Data Type Conversion21/1(In1)  "<1_J>"
  bus_selector1/1 -> Data Type Conversion13/1(In1)  "<polepair>"
  delayMatch/1 -> Product4/1(In1)
  mechanical_system_out1/1 -> Switch11/1
  integrator_out1/1 -> mechanical_system_out1/1
  delayMatch45/1 -> Sum310/2(In2)
  Sum3_outbuff10/1 -> reset_in10/3
  Gain_outbuff9/1 -> Sum310/1(In1)
  Product11_outbuff/1 -> Gain10/2(In2)
  Sum1_outbuff1/1 -> Product11/2(In2)
  Initial_Val10/1 -> reset_in10/1, reset_out10/1
  Product10_outbuff/1 -> Product/1(In1), Product1/1(In1)
  Sum1_stage3_outbuff/1 -> Gain9/2(In2)
  Gain_outbuff8/1 -> Sum39/1(In1)
  Sum3_outbuff9/1 -> reset_in9/3
  Initial_Val9/1 -> reset_in9/1, reset_out9/1
  delayMatch4/1 -> Product6/1(In1)
  delayMatch11/1 -> Product2/2(In2)
  Product2_outbuff/1 -> Sum38/2(In2)
  Sum3_outbuff8/1 -> Factor/2(In2)
  delayMatch10/1 -> Product3/1(In1)
  delayMatch5/1 -> Product1/2(In2)
  Sum2_outbuff1/1 -> Product5/2(In2)
  Product5_outbuff/1 -> i_d/1, Product8/1(In1)
  i_d/1 -> mux/1, Product2/1(In1)
  mux/1 -> Data Type Conversion3/1(In1)
  delayMatch19/1 -> mux/2
  Product6_outbuff/1 -> i_q/1, Product7/1(In1)
  Goto32/1 -> From14/1, From18/1, From22/1, From26/1, From30/1, From4/1, From8/1
  Add1_outbuff/1 -> Gain8/2(In2)
  Gain_outbuff7/1 -> Sum37/1(In1)
  Sum3_outbuff7/1 -> reset_in8/3
  Initial_Val8/1 -> reset_in8/1, reset_out8/1
  delayMatch13/1 -> Divide3/1(In1)
  Divide3_outbuff/1 -> delayMatch21/1, Divide2/2(In2)
  From12/1 -> Divide3/2(In2)
  Goto10/1 -> From12/1
  bus_selector/12 -> Data Type Conversion31/1(In1)  "<L_z3>"
  bus_selector/11 -> Data Type Conversion12/1(In1)  "<L_y2>"
  bus_selector/10 -> Data Type Conversion11/1(In1)  "<L_x2>"
  bus_selector/9 -> Data Type Conversion10/1(In1)  "<L_y1>"
  bus_selector/8 -> Data Type Conversion9/1(In1)  "<L_x1>"
  bus_selector/7 -> Data Type Conversion8/1(In1)  "<L_z2>"
  bus_selector/6 -> Data Type Conversion7/1(In1)  "<L_z1>"
  bus_selector/5 -> Data Type Conversion61/1(In1)  "<psi_pm>"
  bus_selector/4 -> Data Type Conversion51/1(In1)  "<polepair>"
  bus_selector/3 -> Data Type Conversion41/1(In1)  "<R_1>"
  bus_selector/2 -> Data Type Conversion2/1(In1)  "<1_L_q>"
  bus_selector/1 -> Data Type Conversion1/1(In1)  "<1_L_d>"
  Goto9/1 -> From11/1
  From11/1 -> Divide1/2(In2)
  Divide1_outbuff/1 -> delayMatch20/1, Divide/2(In2)
  Add_outbuff/1 -> Gain7/2(In2)
  Gain_outbuff6/1 -> Sum36/1(In1)
  Sum3_outbuff6/1 -> reset_in7/3
  Initial_Val7/1 -> reset_in7/1, reset_out7/1
  Goto1/1 -> From15/1, From19/1, From2/1, From23/1, From27/1, From3/1, From31/1, From5/1, From9/1
  delayMatch18/1 -> Divide13/1(In1)
  Divide13_outbuff/1 -> delayMatch26/1, Divide12/2(In2)
  From21/1 -> Divide13/2(In2)
  Goto15/1 -> From21/1
  Add6_outbuff/1 -> Gain1/2(In2)
  Add5_outbuff/1 -> Gain6/2(In2)
  Gain_outbuff5/1 -> Sum35/1(In1)
  Sum3_outbuff5/1 -> reset_in6/3
  Initial_Val6/1 -> reset_in6/1, reset_out5/1
  delayMatch17/1 -> Divide11/1(In1)
  Divide11_outbuff/1 -> delayMatch25/1, Divide10/2(In2)
  From20/1 -> Divide11/2(In2)
  Goto14/1 -> From20/1
  delayMatch25/1 -> mux/8
  Add4_outbuff/1 -> Gain5/2(In2)
  Gain_outbuff4/1 -> Sum34/1(In1)
  Sum3_outbuff4/1 -> reset_in5/3
  Initial_Val5/1 -> reset_in5/1, reset_out4/1
  delayMatch16/1 -> Divide9/1(In1)
  Divide9_outbuff/1 -> delayMatch24/1, Divide8/2(In2)
  From17/1 -> Divide9/2(In2)
  Goto13/1 -> From17/1
  delayMatch24/1 -> mux/7
  Add3_outbuff/1 -> Gain4/2(In2)
  Gain_outbuff3/1 -> Sum33/1(In1)
  Sum3_outbuff3/1 -> reset_in4/3
  Initial_Val4/1 -> reset_in4/1, reset_out3/1
  delayMatch15/1 -> Divide7/1(In1)
  Divide7_outbuff/1 -> delayMatch23/1, Divide6/2(In2)
  From16/1 -> Divide7/2(In2)
  Goto12/1 -> From16/1
  delayMatch23/1 -> mux/6
  Add2_outbuff/1 -> Gain3/2(In2)
  Gain_outbuff2/1 -> Sum32/1(In1)
  Sum3_outbuff2/1 -> reset_in3/3
  Initial_Val3/1 -> reset_in3/1, reset_out2/1
  delayMatch14/1 -> Divide5/1(In1)
  Divide5_outbuff/1 -> delayMatch22/1, Divide4/2(In2)
  From13/1 -> Divide5/2(In2)
  Goto11/1 -> From13/1
  delayMatch22/1 -> mux/5
  Sum_stage3_outbuff/1 -> Gain2/2(In2)
  Gain_outbuff1/1 -> Sum31/1(In1)
  Sum3_outbuff1/1 -> reset_in2/3
  Initial_Val2/1 -> reset_in2/1, reset_out1/1
  Gain_outbuff/1 -> Sum3/1(In1)
  Sum3_outbuff/1 -> reset_in1/3
  Initial_Val1/1 -> reset_in1/1, reset_out6/1
  delayMatch26/1 -> mux/9
  delayMatch12/1 -> Divide1/1(In1)
  delayMatch20/1 -> mux/3
  Goto33/1 -> From24/1
  From24/1 -> Sum21/2(In2)
  Goto34/1 -> From6/1
  From6/1 -> Product10/2(In2)
  Goto35/1 -> From7/1
  From7/1 -> Product6/2(In2)
  Goto36/1 -> From10/1
  delayMatch9/1 -> Product5/1(In1)
  delayMatch21/1 -> mux/4
  Factor_outbuff/1 -> Product9/1(In1)
  Product9_outbuff/1 -> M_Mi1/1
  Sum2_outbuff/1 -> Switch1/1
  Constant/1 -> Sum1/2(In2), Sum2/1(In1)
  Sum1_outbuff/1 -> Switch/1
  Switch1/1 -> reset_in/3
  Initial_Val/1 -> reset_in/1, reset_out/1
  delayMatch1/1 -> Sum/1(In1)
  delayMatch50/1 -> currents_dq_output/1
  delayMatch49/1 -> theta_el/1
  in15_repeat/1 -> reset_out10/3
  in13_repeat/1 -> delayMatch44/1
  in12_repeat/1 -> reset_out9/3
  in11_repeat/1 -> reset_out8/3
  in10_repeat/1 -> bus_selector/1, bus_selector1/1
  in9_repeat/1 -> reset_out7/3
  in8_repeat/1 -> reset_out6/3
  in6_repeat/1 -> reset_out5/3
  in5_repeat/1 -> reset_out4/3
  in4_repeat/1 -> reset_out3/3
  in3_repeat/1 -> reset_out2/3
  in2_repeat/1 -> reset_out1/3
  in1_repeat/1 -> reset_out/3
  crp_out_delay13/1 -> Delay1_lowered10/1
  crp_out_delay12/1 -> Delay1_lowered9/1
  crp_out_delay11/1 -> Delay1_lowered8/1
  crp_out_delay10/1 -> Delay1_lowered7/1
  crp_out_delay9/1 -> Delay1_lowered6/1
  crp_out_delay8/1 -> Delay1_lowered5/1
  crp_out_delay7/1 -> Delay1_lowered4/1
  crp_out_delay6/1 -> Delay1_lowered3/1
  crp_out_delay5/1 -> Delay1_lowered2/1
  crp_out_delay4/1 -> Delay2/1
  crp_out_delay3/1 -> Delay1/1
  crp_out_delay2/1 -> Delay1_lowered1/1
  crp_out_delay1/1 -> Delay/1
  crp_out_delay/1 -> Delay1_lowered/1
  Delay1_lowered10/1 -> in15_repeat/1
  Delay1_lowered9/1 -> in6_repeat/1
  Delay1_lowered8/1 -> in5_repeat/1
  Delay1_lowered7/1 -> in4_repeat/1
  Delay1_lowered6/1 -> in3_repeat/1
  Delay1_lowered5/1 -> in2_repeat/1
  Delay1_lowered4/1 -> in8_repeat/1
  Delay1_lowered3/1 -> in9_repeat/1
  Delay1_lowered2/1 -> in11_repeat/1
  Delay2/1 -> in13_repeat/1
  Delay1_lowered1/1 -> in12_repeat/1
  Delay1_lowered/1 -> in1_repeat/1
  physical_parameters/1 -> in10_repeat/1
  voltage_input_dq/1 -> Data Type Conversion/1(In1)
  omega_mech/1 -> Switch11/3
  <simulate_mechanical>/1 -> Switch11/2
  <reset_integrators>/1 -> in0_buff/1
  load_torque/1 -> Data Type Conversion71/1(In1)
  Delay/1 -> omega_out/1
  Delay1/1 -> M_Mi/1

== system gm_uz_pmsm_model_9ph_21b_all_double_vnl/uz_pmsm_model_9ph_vnl/Line-Line to Phase voltage ==
  In1 : Inport
  Complex to Real-Imag : ComplexToRealImag
  Constant : Constant  Value=0  OutDataTypeStr=fixdt(1,25,12)  SampleTime=ts
  Constant1 : Constant  Value=1/sqrt(3)*exp(1i*-30/180*pi)  OutDataTypeStr=fixdt(1,18,16)  SampleTime=ts
  Demux3 : Demux  Outputs=3
  Mux4 : Mux  Inputs=3
  Product : Product  OutDataTypeStr=fixdt(1,25,12)
  Real-Imag to Complex : RealImagToComplex
  Terminator : Terminator
  abc   to   alpha_beta_0 : Subsystem
  alpha_beta_0   to   abc : Subsystem
  Out1 : Outport
  wires:
  Constant1/1 -> Product/2
  alpha_beta_0   to   abc/1("a, b, c") -> Out1/1
  abc   to   alpha_beta_0/1("alpha, beta, 0 ") -> Demux3/1
  Demux3/3 -> Terminator/1
  In1/1 -> abc   to   alpha_beta_0/1("a, b, c")
  Constant/1 -> Mux4/3
  Complex to Real-Imag/2 -> Mux4/2
  Demux3/1 -> Real-Imag to Complex/1
  Real-Imag to Complex/1 -> Product/1
  Product/1 -> Complex to Real-Imag/1
  Mux4/1 -> alpha_beta_0   to   abc/1("alpha, beta, 0  ")
  Complex to Real-Imag/1 -> Mux4/1
  Demux3/2 -> Real-Imag to Complex/2

== system gm_uz_pmsm_model_9ph_21b_all_double_vnl/uz_pmsm_model_9ph_vnl/Line-Line to Phase voltage1 ==
  In1 : Inport
  Complex to Real-Imag : ComplexToRealImag
  Constant : Constant  Value=0  OutDataTypeStr=fixdt(1,25,12)  SampleTime=ts
  Constant1 : Constant  Value=1/sqrt(3)*exp(1i*-30/180*pi)  OutDataTypeStr=fixdt(1,18,16)  SampleTime=ts
  Demux3 : Demux  Outputs=3
  Mux4 : Mux  Inputs=3
  Product : Product  OutDataTypeStr=fixdt(1,25,12)
  Real-Imag to Complex : RealImagToComplex
  Terminator : Terminator
  abc   to   alpha_beta_0 : Subsystem
  alpha_beta_0   to   abc : Subsystem
  Out1 : Outport
  wires:
  Demux3/2 -> Real-Imag to Complex/2
  Complex to Real-Imag/1 -> Mux4/1
  Mux4/1 -> alpha_beta_0   to   abc/1("alpha, beta, 0  ")
  Product/1 -> Complex to Real-Imag/1
  Real-Imag to Complex/1 -> Product/1
  Demux3/1 -> Real-Imag to Complex/1
  Complex to Real-Imag/2 -> Mux4/2
  Constant/1 -> Mux4/3
  In1/1 -> abc   to   alpha_beta_0/1("a, b, c")
  Demux3/3 -> Terminator/1
  abc   to   alpha_beta_0/1("alpha, beta, 0 ") -> Demux3/1
  alpha_beta_0   to   abc/1("a, b, c") -> Out1/1
  Constant1/1 -> Product/2

== system gm_uz_pmsm_model_9ph_21b_all_double_vnl/uz_pmsm_model_9ph_vnl/Line-Line to Phase voltage2 ==
  In1 : Inport
  Complex to Real-Imag : ComplexToRealImag
  Constant : Constant  Value=0  OutDataTypeStr=fixdt(1,25,12)  SampleTime=ts
  Constant1 : Constant  Value=1/sqrt(3)*exp(1i*-30/180*pi)  OutDataTypeStr=fixdt(1,18,16)  SampleTime=ts
  Demux3 : Demux  Outputs=3
  Mux4 : Mux  Inputs=3
  Product : Product  OutDataTypeStr=fixdt(1,25,12)
  Real-Imag to Complex : RealImagToComplex
  Terminator : Terminator
  abc   to   alpha_beta_0 : Subsystem
  alpha_beta_0   to   abc : Subsystem
  Out1 : Outport
  wires:
  Constant1/1 -> Product/2
  alpha_beta_0   to   abc/1("a, b, c") -> Out1/1
  abc   to   alpha_beta_0/1("alpha, beta, 0 ") -> Demux3/1
  Demux3/3 -> Terminator/1
  In1/1 -> abc   to   alpha_beta_0/1("a, b, c")
  Constant/1 -> Mux4/3
  Complex to Real-Imag/2 -> Mux4/2
  Demux3/1 -> Real-Imag to Complex/1
  Real-Imag to Complex/1 -> Product/1
  Product/1 -> Complex to Real-Imag/1
  Mux4/1 -> alpha_beta_0   to   abc/1("alpha, beta, 0  ")
  Complex to Real-Imag/1 -> Mux4/1
  Demux3/2 -> Real-Imag to Complex/2

== system gm_uz_pmsm_model_9ph_21b_all_double_vnl/uz_pmsm_model_9ph_vnl/Transformation ==
  in : Inport
  Add : Sum
  Add1 : Sum  Inputs=-+
  Constant1 : Constant  Value=c  OutDataTypeStr=fixdt(1,18,17)  SampleTime=ts
  Data Type Conversion39 : DataTypeConversion  OutDataTypeStr=single  RndMeth=Nearest
  Demux1 : Demux  Outputs=9
  Divide{,1..3} (4 alike) : Product  Inputs=**
  MatrixMultiply : Product  Multiplication=Matrix(*)  OutDataTypeStr=fixdt(1,25,12)
  Mux : Mux  Inputs=9
  out : Outport
  wires:
  in/1 -> MatrixMultiply/2
  Data Type Conversion39/1 -> Demux1/1
  Constant1/1 -> MatrixMultiply/1
  MatrixMultiply/1 -> Data Type Conversion39/1
  Divide2/1 -> Add1/1
  Divide3/1 -> Add1/2
  [cos_theta_el] -> Divide3/1
  [sin_theta_el] -> Divide2/1
  [cos_theta_el] -> Divide/1  "cos_theta_hdl"
  [sin_theta_el] -> Divide1/1  "sin_theta_hdl"
  Divide1/1 -> Add/2
  Divide/1 -> Add/1
  Demux1/2 -> Divide3/2, Divide1/2  "u_beta"
  Demux1/1 -> Divide2/2, Divide/2  "u_alpha"
  Add/1 -> Mux/1
  Add1/1 -> Mux/2
  Mux/1 -> out/1  "trafo_out"
  Demux1/9 -> Mux/9
  Demux1/8 -> Mux/8
  Demux1/7 -> Mux/7
  Demux1/6 -> Mux/6
  Demux1/5 -> Mux/5
  Demux1/4 -> Mux/4
  Demux1/3 -> Mux/3

== system gm_uz_pmsm_model_9ph_21b_all_double_vnl/uz_pmsm_model_9ph_vnl/Transformation1 ==
  in : Inport
  Add : Sum  Inputs=+-
  Add1 : Sum
  Constant1 : Constant  Value=inv(c)  OutDataTypeStr=fixdt(1,18,16)  SampleTime=ts
  Data Type Conversion28 : DataTypeConversion  OutDataTypeStr=fixdt(1,25,12)  RndMeth=Nearest
  Demux1 : Demux  Outputs=9
  Divide{,1..3} (4 alike) : Product  Inputs=**
  MatrixMultiply : Product  Multiplication=Matrix(*)  OutDataTypeStr=fixdt(1,25,12)
  Mux : Mux  Inputs=9
  out : Outport
  wires:
  MatrixMultiply/1 -> out/1
  Constant1/1 -> MatrixMultiply/1
  Data Type Conversion28/1 -> MatrixMultiply/2
  Add1/1 -> Mux/2
  [cos_theta_el] -> Divide3/1
  Divide2/1 -> Add1/1
  [sin_theta_el] -> Divide2/1
  Divide3/1 -> Add1/2
  Demux1/1 -> Divide/2, Divide2/2  "i_d"
  Divide1/1 -> Add/2
  [cos_theta_el] -> Divide/1
  Divide/1 -> Add/1
  Add/1 -> Mux/1
  Demux1/2 -> Divide1/2, Divide3/2  "i_q"
  [sin_theta_el] -> Divide1/1
  Demux1/7 -> Mux/7
  Demux1/9 -> Mux/9
  Demux1/5 -> Mux/5
  Demux1/3 -> Mux/3
  Demux1/4 -> Mux/4
  Demux1/6 -> Mux/6
  Demux1/8 -> Mux/8
  Mux/1 -> Data Type Conversion28/1
  in/1 -> Demux1/1

== system gm_uz_pmsm_model_9ph_21b_all_double_vnl/uz_pmsm_model_9ph_vnl/dq_model_9ph ==
  note: Mechanical
  note: PMSM electric and magentic
  note: This signal introduces an algebraic loop if simulate_mechanical is true!
  load_torque : Inport
  <reset_integrators> : Inport  Port=2
  <simulate_mechanical> : Inport  Port=3
  omega_mech : Inport  Port=4
  voltage_input_dq : Inport  Port=5
  physical_parameters : Inport  Port=6
  Bus Selector : BusSelector  OutputSignals=polepair,1_J
  Data Type Conversion{,1..2,7} (4 alike) : DataTypeConversion  OutDataTypeStr=double  RndMeth=Nearest
  Data Type Conversion{3..6} (4 alike) : DataTypeConversion  OutDataTypeStr=single  RndMeth=Nearest
  Delay : Delay  DelayLength=1
  Delay1 : Delay  DelayLength=1
  Demux : Demux  Outputs=9
  Mux : Mux  Inputs=9
  Switch1 : Switch  Criteria=u2 ~= 0
  Wrapped State DTI : Subsystem
  mechanical_system : Subsystem
  pmsm : Subsystem
  torque_calculation : Subsystem
  theta_el : Outport
  currents_dq_output : Outport  Port=2
  M_Mi : Outport  Port=3
  omega_out : Outport  Port=4
  wires:
  Data Type Conversion7/1 -> mechanical_system/4(load_torque)
  Wrapped State DTI/1(Angular Position) -> Data Type Conversion6/1  "theta_el"
  Data Type Conversion6/1 -> theta_el/1
  Data Type Conversion5/1 -> Delay/1
  Data Type Conversion4/1 -> Delay1/1
  Data Type Conversion3/1 -> currents_dq_output/1
  Data Type Conversion2/1 -> mechanical_system/3(reciprocal_J)
  Data Type Conversion1/1 -> Wrapped State DTI/2(polepair), torque_calculation/5(polepairs)
  physical_parameters/1 -> pmsm/12(physical_parameters), Bus Selector/1
  Data Type Conversion/1 -> Demux/1
  Delay1/1 -> M_Mi/1
  Delay/1 -> omega_out/1
  Bus Selector/2 -> Data Type Conversion2/1  "<1_J>"
  Bus Selector/1 -> Data Type Conversion1/1  "<polepair>"
  Mux/1 -> Data Type Conversion3/1
  pmsm/8(i_y1) -> Mux/6  "i_y1"
  Switch1/1 -> Wrapped State DTI/1(Angular Speed), Data Type Conversion5/1, pmsm/11(omega_mech)
  load_torque/1 -> Data Type Conversion7/1
  mechanical_system/1(omega_mech) -> Switch1/1
  pmsm/4(I_q) -> Mux/2, torque_calculation/2(I_q)  "i_q"
  <reset_integrators>/1 -> pmsm/1(reset), mechanical_system/1(reset), Wrapped State DTI/3(reset)
  pmsm/5(i_o1) -> Mux/3  "i_o1"
  Demux/6 -> pmsm/7(u_y1)
  <simulate_mechanical>/1 -> Switch1/2
  pmsm/2(psi_q) -> torque_calculation/4(psi_q)
  omega_mech/1 -> Switch1/3
  pmsm/1(psi_d) -> torque_calculation/3(psi_d)
  Demux/8 -> pmsm/9(u_y2)
  torque_calculation/1(M_Mi) -> mechanical_system/2(M_Mi), Data Type Conversion4/1
  pmsm/10(i_y2) -> Mux/8  "i_y2"
  voltage_input_dq/1 -> Data Type Conversion/1
  pmsm/7(i_x1) -> Mux/5  "i_x1"
  pmsm/9(i_x2) -> Mux/7  "i_x2"
  Demux/9 -> pmsm/10(u_zero)
  Demux/2 -> pmsm/3(u_q)  "u_q"
  Demux/4 -> pmsm/5(u_o2)
  pmsm/6(i_o2) -> Mux/4  "i_o2"
  pmsm/11(i_zero) -> Mux/9  "i_zero"
  Demux/1 -> pmsm/2(u_d)  "u_d"
  pmsm/3(I_d) -> Mux/1, torque_calculation/1(I_d)  "i_d"
  Demux/3 -> pmsm/4(u_o1)
  Demux/7 -> pmsm/8(u_x2)
  Demux/5 -> pmsm/6(u_x1)

== system gm_uz_pmsm_model_9ph_21b_all_double_vnl/Compare/Assert_i_abc_ps/RelErrCheck ==
  In1 : Inport
  In2 : Inport  Port=2
  "RelativeErrorCheck " : MATLAB Function  TreatAsAtomicUnit=on
  Out1 : Outport  VectorParamsAs1DForOutWhenUnconnected=off
  wires:
  "RelativeErrorCheck "/1(y) -> Out1/1
  In1/1 -> "RelativeErrorCheck "/1(P)
  In2/1 -> "RelativeErrorCheck "/2(R)

== system gm_uz_pmsm_model_9ph_21b_all_double_vnl/Compare/Assert_outputs/RelErrCheck ==
  In1 : Inport
  In2 : Inport  Port=2
  "RelativeErrorCheck " : MATLAB Function  TreatAsAtomicUnit=on
  Out1 : Outport  VectorParamsAs1DForOutWhenUnconnected=off
  wires:
  "RelativeErrorCheck "/1(y) -> Out1/1
  In1/1 -> "RelativeErrorCheck "/1(P)
  In2/1 -> "RelativeErrorCheck "/2(R)
